simulink model "Long_Transmission_Line"  (R2020a)
settings: Solver=VariableStepAuto  StartTime=0.0  StopTime=1  RelTol=1e-3
libraries: powerlib x6, powerlib_meascontrol x6
settings Model: Creator=Reaga  LastModifiedBy=Reaga

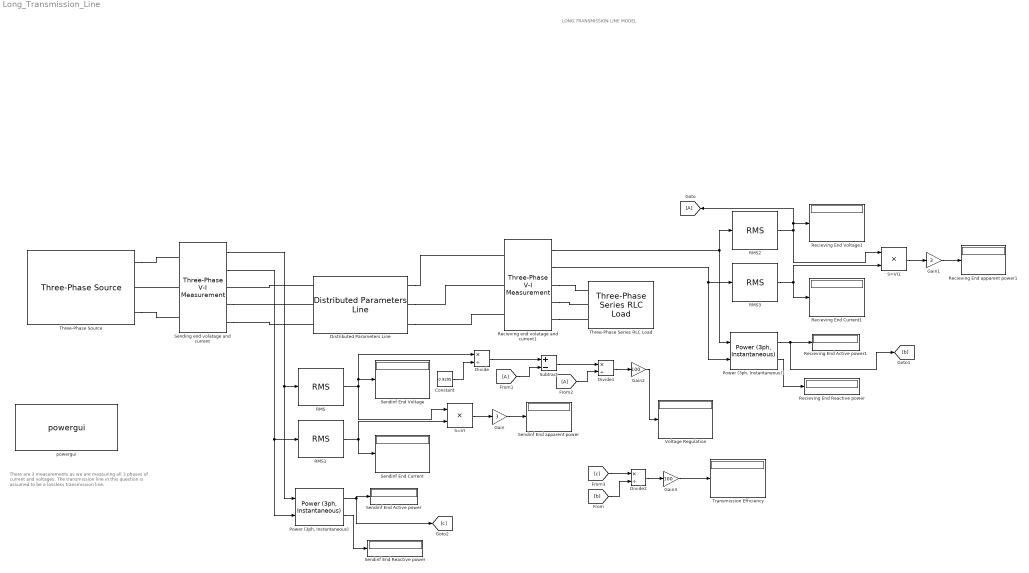
== system Long_Transmission_Line ==
  note: There are 3 measurements as we are measuring all 3 phases
      | of current and voltages.
      |
      | The transmission line in this question is assumed to be a lossless transmission line.
  note: LONG TRANSMISSION LINE MODEL
  Constant : Constant  Value=0.9295
  Distributed Parameters Line : powerlib/Elements/Distributed Parameters Line  Phases=3  Frequency=60  Resistance=[0 0]  Inductance="[0.97e-3  0.99e-3]"  Capacitance=[11.5e-9 11.5e-9]  Length=300  x1=[5.82076609134674e-11 617530 617530;376.991118430775 376.991118430775 376.991118430775;1.18918707880175 0.426861843081656 -1.14393448371324]  x2=[4.36557456851006e-11 499987.196622057 499987.196622057;376.991118430775 376.991118430775 376.991118430775;-0.38160924799315 0.145647927793821 -1.42514839900108]  x3=[5.91460143700054e-13 1206.114766815 1206.11476681501;376.991118430775 376.991118430775 376.991118430775;2.48003358307285 1.23771807602482 -0.333078250770074]  x4=[8.82447164727866e-13 3531.62978476019 3531.62978476019;376.991118430775 376.991118430775 376.991118430775;-0.121006856245809 -0.201032665608174 -1.77182899240307]  x5=0.00101224996912818  V1=[5.821e-11 6.175e+05 6.175e+05;377 377 377;1.189 0.4269 -1.144]  V2=[4.366e-11 5e+05 5e+05;377 377 377;-0.3816 0.1456 -1.425]  I1=[5.915e-13 1206 1206;377 377 377;2.48 1.238 -0.3331]  I2=[8.824e-13 3532 3532;377 377 377;-0.121 -0.201 -1.772]  nHarmo=1  Measurements=None
  Divide : Product  Inputs=*/
  Divide1 : Product  Inputs=*/
  Divide2 : Product  Inputs=*/
  Gain : Gain  Gain=3
  Gain1 : Gain  Gain=3
  Gain2 : Gain  Gain=100
  Gain3 : Gain  Gain=100
  "Power (3ph, Instantaneous)" : powerlib_meascontrol/Measurements/Power (3ph, Instantaneous)
  "Power (3ph, Instantaneous)1" : powerlib_meascontrol/Measurements/Power (3ph, Instantaneous)
  RMS{,1..3} (4 alike) : powerlib_meascontrol/Measurements/RMS  TrueRMS=on  Freq=60  RMSInit=0  Ts=0
  Recieving End Active power1 : Display
  Recieving End Current1 : Display
  "Recieving End Reactive power " : Display
  Recieving End Voltage1 : Display
  Recieving End apparent power1 : Display
  Recieving end volatage and current1 : powerlib/Measurements/Three-Phase V-I Measurement  VoltageMeasurement=phase-to-ground  SetLabelV=off  LabelV=Vabc  Vpu=off  VpuLL=off  CurrentMeasurement=yes  SetLabelI=off  LabelI=Iabc  Ipu=off  Pbase=100e6  Vbase=500e3  OutputType=Complex  PhasorSimulation=off  PSBequivalent=0
  S=VI : Product
  S=VI1 : Product
  Sendinf End Active power : Display
  Sendinf End Current : Display
  "Sendinf End Reactive power " : Display
  Sendinf End Voltage : Display
  Sendinf End apparent power : Display
  Sending end volatage and current : powerlib/Measurements/Three-Phase V-I Measurement  VoltageMeasurement=phase-to-ground  SetLabelV=off  LabelV=Vabc  Vpu=off  VpuLL=off  CurrentMeasurement=yes  SetLabelI=off  LabelI=Iabc  Ipu=off  Pbase=100e6  Vbase=500e3  OutputType=Complex  PhasorSimulation=off  PSBequivalent=0
  Subtract : Sum  Inputs=+-
  Three-Phase Series RLC Load : powerlib/Elements/Three-Phase Series RLC Load  LConnTagsString=A|B|C  Configuration=Y (grounded)  NominalVoltage=500e3  Vabc=[1e3 1e3 1e3]  Vabcp=[1e3 1e3 1e3]  NominalFrequency=60  UnbalancedPower=off  ActivePower=800e6  InductivePower=600e6  CapacitivePower=0  Pabc=[10e3 9e3 11e3]  QLabc=[100 90 110]  QCabc=[100 90 110]  Pabcp=[10e3 9e3 11e3]  QLabcp=[100 90 110]  QCabcp=[100 90 110]  Measurements=None  LoadType=constant Z
  Three-Phase Source : powerlib/Electrical Sources/Three-Phase Source  InternalConnection=Yg  VoltagePhases=off  Voltage=617.53e3  PhaseAngle=16.1  Voltage_phases=[25e3 25e3 25e3]/sqrt(3)  PhaseAngles_phases=[0 -120 +120]  Frequency=60  NonIdealSource=off  SpecifyImpedance=off  Resistance=0.8929  Inductance=16.58e-3  ShortCircuitLevel=100e6  BaseVoltage=25e3  XRratio=7  BusType=swing  Pref=10e3  Qref=0  Prefabc=[10e3, 10e3, 10e3]  Qrefabc=[0, 0, 0]  Qmin=-inf  Qmax=inf
  Transmission Efficiency : Display
  Voltage Regulation : Display
  powergui : powerlib/powergui  Priority=1  SimulationMode=Continuous  SampleTime=50e-6  frequency=60  Iterations=50  frequencyindice=60  Pbase=100e6  ErrMax=1e-4  UnitsV=kV  UnitsW=MW  buscounter=0  FunctionMessages=off  echomessages=off  EnableUseOfTLC=off  CurrentSourceSwitches=off  DisableSnubberDevices=off  DisableRonSwitches=off  DisableVfSwitches=off  DisplayEquations=off  AutomaticDiscreteSolvers=off  SolverType=Tustin/Backward Euler (TBE)  Interpol=off  ExternalGateDelay=off  methode=off  Ts=100  x0status=blocks  SPID=on  SwTol=0  HookPort=off  NonlinearTolerance=1e-4  nMaxIteration=100  ContinueOnMaxIteration=off  RestoreLinks=warning  ResistiveCurrentMeasurement=off  Frange=[0:2:500]  Ylog=off  Xlog=on  ShowGrid=off  save=off  variable=ZData  structure=0  ZoomFFT=off  StartTime=0.0  cycles=1  DisplayStyle=1  fundamental=60  FreqAxis=off  MaxFrequency=1000  frequencyindicesteady=1  RmsSteady=1  display=off
  wires:
  Sending end volatage and current/1 -> "Power (3ph, Instantaneous)"/1, RMS/1
  RMS/1 -> Divide/1, Sendinf End Voltage/1, S=VI/1
  RMS1/1 -> Sendinf End Current/1, S=VI/2
  Sending end volatage and current/2 -> "Power (3ph, Instantaneous)"/2, RMS1/1
  "Power (3ph, Instantaneous)"/1 -> [c], Sendinf End Active power/1
  "Power (3ph, Instantaneous)"/2 -> "Sendinf End Reactive power "/1
  S=VI/1 -> Gain/1
  Gain/1 -> Sendinf End apparent power/1
  S=VI1/1 -> Gain1/1
  Recieving end volatage and current1/2 -> "Power (3ph, Instantaneous)1"/2, RMS3/1
  RMS2/1 -> [A], Recieving End Voltage1/1, S=VI1/1
  "Power (3ph, Instantaneous)1"/2 -> "Recieving End Reactive power "/1
  Recieving end volatage and current1/1 -> "Power (3ph, Instantaneous)1"/1, RMS2/1
  Gain1/1 -> Recieving End apparent power1/1
  "Power (3ph, Instantaneous)1"/1 -> Recieving End Active power1/1, [b]
  RMS3/1 -> Recieving End Current1/1, S=VI1/2
  Divide/1 -> Subtract/1
  Constant/1 -> Divide/2
  [A] -> Subtract/2
  Subtract/1 -> Divide1/1
  [A] -> Divide1/2
  Divide1/1 -> Gain2/1
  Gain2/1 -> Voltage Regulation/1
  [c] -> Divide2/1
  [b] -> Divide2/2
  Divide2/1 -> Gain3/1
  Gain3/1 -> Transmission Efficiency/1
  connections:
  Sending end volatage and current/LConn2 -- Three-Phase Source/RConn2
  Three-Phase Source/RConn1 -- Sending end volatage and current/LConn1
  Three-Phase Source/RConn3 -- Sending end volatage and current/LConn3
  Distributed Parameters Line/LConn1 -- Sending end volatage and current/RConn1
  Sending end volatage and current/RConn2 -- Distributed Parameters Line/LConn2
  Sending end volatage and current/RConn3 -- Distributed Parameters Line/LConn3
  Distributed Parameters Line/RConn3 -- Recieving end volatage and current1/LConn3
  Distributed Parameters Line/RConn2 -- Recieving end volatage and current1/LConn2
  Distributed Parameters Line/RConn1 -- Recieving end volatage and current1/LConn1
  Recieving end volatage and current1/RConn1 -- Three-Phase Series RLC Load/LConn1
  Recieving end volatage and current1/RConn2 -- Three-Phase Series RLC Load/LConn2
  Recieving end volatage and current1/RConn3 -- Three-Phase Series RLC Load/LConn3
